simulink model "MRAC_OutputFeedback_Tau"  (R2017b)
settings: Solver=VariableStepAuto  StartTime=0.0  StopTime=100  RelTol=1e-3
values from neighbouring files (symbols this model uses):
  Ix = 0.0552    [ProportionalController.m]    (also in discrete1.m; discrete2.m; istr.m; proportionalTest.m = 0.0235)
  Iy = 0.0552    [ProportionalController.m]    (also in discrete1.m; discrete2.m; istr.m; proportionalTest.m = 0.0494)
  Iz = 0.11    [ProportionalController.m]    (also in discrete1.m; discrete2.m; istr.m; proportionalTest.m = 0.6121)
  wn = 4/(zeta*Ts)    [SecondOrderResponse.m]
  zeta = 0.7    [RLS_demo_init.m]    (also in SecondOrderResponse.m = sqrt(A/(pi^2+A)))
undefined symbols (not defined in the file or in its folder): a0, b0_zero_p, b0_zero_r, b0_zero_y, DiscIntNeverNeededParam, gamma1_p, gamma1_r, gamma1_y, gamma2_p, gamma2_r, gamma2_y, theta_zero_p, theta_zero_r, theta_zero_y
libraries: simulink_extras x15
settings Model: Creator=YvesDaoud  LastModifiedBy=YvesDaoud

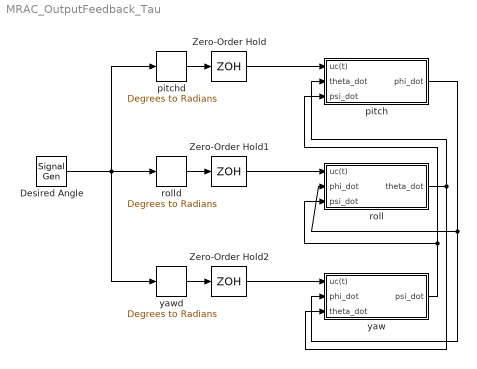
== system MRAC_OutputFeedback_Tau ==
  Desired Angle : SignalGenerator  WaveForm=square  Amplitude=5  Frequency=0.05
  Zero-Order Hold : ZeroOrderHold  SampleTime=1/2000
  Zero-Order Hold1 : ZeroOrderHold  SampleTime=1/2000
  Zero-Order Hold2 : ZeroOrderHold  SampleTime=1/2000
  pitch : Subsystem
  pitchd : simulink_extras/Transformations/Degrees to Radians
  roll : Subsystem
  rolld : simulink_extras/Transformations/Degrees to Radians
  yaw : Subsystem
  yawd : simulink_extras/Transformations/Degrees to Radians
  wires:
  rolld/1 -> Zero-Order Hold1/1
  yawd/1 -> Zero-Order Hold2/1
  Zero-Order Hold/1 -> pitch/1(uc(t))
  Zero-Order Hold1/1 -> roll/1(uc(t))
  Desired Angle/1 -> pitchd/1, yawd/1, rolld/1
  pitchd/1 -> Zero-Order Hold/1
  Zero-Order Hold2/1 -> yaw/1(uc(t))
  roll/1(theta_dot) -> yaw/3(theta_dot), pitch/2(theta_dot)
  pitch/1(phi_dot) -> roll/2(phi_dot), yaw/2(phi_dot)
  yaw/1(psi_dot) -> roll/3(psi_dot), pitch/3(psi_dot)

== system MRAC_OutputFeedback_Tau/pitch ==
  uc(t) : Inport
  theta_dot : Inport  Port=2
  psi_dot : Inport  Port=3
  Controller : Subsystem
  Plant : Subsystem
  Plotting : Subsystem
  Reference Model : Subsystem
  augmented error : Subsystem
  b0_hat : Subsystem
  eta n : Subsystem
  theta : Subsystem
  phi_dot : Outport
  wires:
  Plant/1(y(t)) -> Plotting/2(y(t)), theta/3(y(t)), Controller/2(y(t)), augmented error/1(y(t)), eta n/2(y(t))
  Reference Model/1(ym(t)) -> Plotting/3(ym(t)), augmented error/2(ym(t))
  Controller/1(u(t)) -> Plant/1(u(t)), Plotting/4(u(t)), eta n/1(u(t)), theta/2(u(t))
  theta/1(theta) -> Controller/3(theta), eta n/4(theta)
  eta n/1(eta n) -> b0_hat/1(eta n), augmented error/4(eta n)
  b0_hat/1(b0_hat) -> Plotting/5(b0_hat), augmented error/3(b0_hat)
  uc(t)/1 -> Plotting/1(uc(t)), theta/4(uc(t)), Reference Model/1(uc(t)), eta n/3(uc(t)), Controller/1(uc(t))
  augmented error/1(epsilon) -> b0_hat/2(epsilon), theta/1(epsilon)
  theta_dot/1 -> Plant/2(theta_dot)
  psi_dot/1 -> Plant/3(psi_dot)
  Plant/2(y_dot(t)) -> phi_dot/1

== system MRAC_OutputFeedback_Tau/roll ==
  uc(t) : Inport
  phi_dot : Inport  Port=2
  psi_dot : Inport  Port=3
  Controller : Subsystem
  Plant : Subsystem
  Plotting : Subsystem
  Reference Model : Subsystem
  augmented error : Subsystem
  b0_hat : Subsystem
  eta n : Subsystem
  theta : Subsystem
  theta_dot : Outport
  wires:
  Plant/2(y_dot(t)) -> theta_dot/1
  psi_dot/1 -> Plant/3(psi_dot)
  phi_dot/1 -> Plant/2(phi_dot)
  augmented error/1(epsilon) -> theta/1(epsilon), b0_hat/2(epsilon)
  uc(t)/1 -> Controller/1(uc(t)), eta n/3(uc(t)), Reference Model/1(uc(t)), theta/4(uc(t)), Plotting/1(uc(t))
  b0_hat/1(b0_hat) -> augmented error/3(b0_hat), Plotting/5(b0_hat)
  eta n/1(eta n) -> augmented error/4(eta n), b0_hat/1(eta n)
  theta/1(theta) -> eta n/4(theta), Controller/3(theta)
  Controller/1(u(t)) -> theta/2(u(t)), eta n/1(u(t)), Plotting/4(u(t)), Plant/1(u(t))
  Reference Model/1(ym(t)) -> augmented error/2(ym(t)), Plotting/3(ym(t))
  Plant/1(y(t)) -> eta n/2(y(t)), augmented error/1(y(t)), Controller/2(y(t)), theta/3(y(t)), Plotting/2(y(t))

== system MRAC_OutputFeedback_Tau/yaw ==
  uc(t) : Inport
  phi_dot : Inport  Port=2
  theta_dot : Inport  Port=3
  Controller : Subsystem
  Plant : Subsystem
  Plotting : Subsystem
  Reference Model : Subsystem
  augmented error : Subsystem
  b0_hat : Subsystem
  eta n : Subsystem
  theta : Subsystem
  psi_dot : Outport
  wires:
  Plant/1(y(t)) -> Plotting/2(y(t)), theta/3(y(t)), Controller/2(y(t)), augmented error/1(y(t)), eta n/2(y(t))
  Reference Model/1(ym(t)) -> Plotting/3(ym(t)), augmented error/2(ym(t))
  Controller/1(u(t)) -> Plant/1(u(t)), Plotting/4(u(t)), eta n/1(u(t)), theta/2(u(t))
  theta/1(theta) -> Controller/3(theta), eta n/4(theta)
  eta n/1(eta n) -> b0_hat/1(eta n), augmented error/4(eta n)
  b0_hat/1(b0_hat) -> Plotting/5(b0_hat), augmented error/3(b0_hat)
  uc(t)/1 -> Plotting/1(uc(t)), theta/4(uc(t)), Reference Model/1(uc(t)), eta n/3(uc(t)), Controller/1(uc(t))
  augmented error/1(epsilon) -> b0_hat/2(epsilon), theta/1(epsilon)
  phi_dot/1 -> Plant/2(phi_dot)
  theta_dot/1 -> Plant/3(theta_dot)
  Plant/2(y_dot(t)) -> psi_dot/1

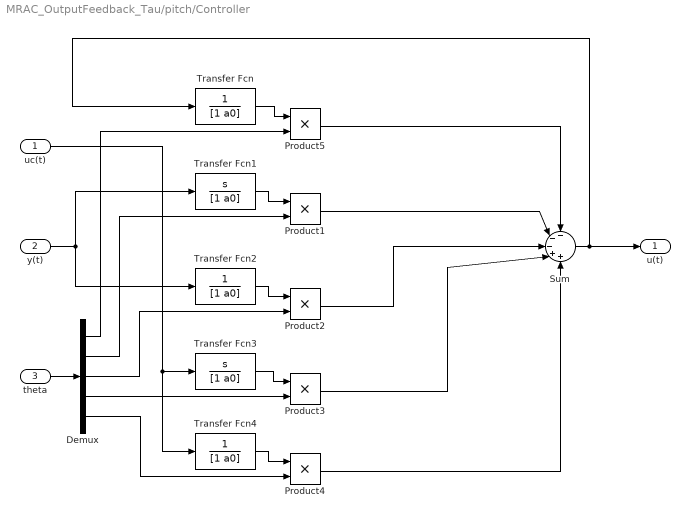
== system MRAC_OutputFeedback_Tau/pitch/Controller ==
  uc(t) : Inport
  y(t) : Inport  Port=2
  theta : Inport  Port=3
  Demux : Demux  Outputs=5
  Product{1..5} (5 alike) : Product
  Sum : Sum  Inputs=---++
  Transfer Fcn : TransferFcn  Denominator=[1 a0]
  Transfer Fcn1 : TransferFcn  Numerator=[1 0]  Denominator=[1 a0]
  Transfer Fcn2 : TransferFcn  Denominator=[1 a0]
  Transfer Fcn3 : TransferFcn  Numerator=[1 0]  Denominator=[1 a0]
  Transfer Fcn4 : TransferFcn  Denominator=[1 a0]
  u(t) : Outport
  wires:
  theta/1 -> Demux/1
  Transfer Fcn1/1 -> Product1/1
  Transfer Fcn2/1 -> Product2/1
  Transfer Fcn3/1 -> Product3/1
  Transfer Fcn4/1 -> Product4/1
  Transfer Fcn/1 -> Product5/1
  Sum/1 -> u(t)/1, Transfer Fcn/1
  Demux/1 -> Product5/2
  Product5/1 -> Sum/1
  Product1/1 -> Sum/2
  Product2/1 -> Sum/3
  Product3/1 -> Sum/4
  Product4/1 -> Sum/5
  y(t)/1 -> Transfer Fcn2/1, Transfer Fcn1/1
  Demux/2 -> Product1/2
  Demux/3 -> Product2/2
  Demux/4 -> Product3/2
  uc(t)/1 -> Transfer Fcn4/1, Transfer Fcn3/1
  Demux/5 -> Product4/2

== system MRAC_OutputFeedback_Tau/pitch/Plant ==
  u(t) : Inport
  theta_dot : Inport  Port=2
  psi_dot : Inport  Port=3
  Constant : Constant  Value=(Iy-Iz)/Ix
  Constant1 : Constant  Value=1/Ix
  Integrator : Integrator
  Integrator1 : Integrator
  Product : Product  Inputs=3
  Product1 : Product
  Sum : Sum  Inputs=+|+
  y(t) : Outport
  y_dot(t) : Outport  Port=2
  wires:
  u(t)/1 -> Product1/1
  Integrator/1 -> y_dot(t)/1, Integrator1/1
  Integrator1/1 -> y(t)/1
  theta_dot/1 -> Product/2
  Product1/1 -> Sum/1
  Constant1/1 -> Product1/2
  Constant/1 -> Product/1
  Product/1 -> Sum/2
  Sum/1 -> Integrator/1
  psi_dot/1 -> Product/3

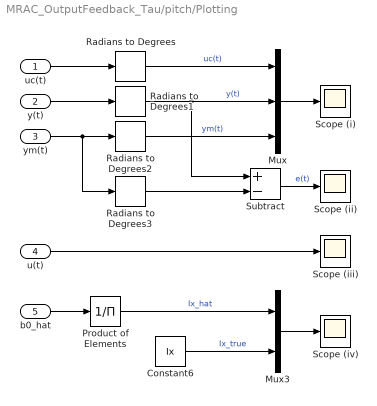
== system MRAC_OutputFeedback_Tau/pitch/Plotting ==
  uc(t) : Inport
  y(t) : Inport  Port=2
  ym(t) : Inport  Port=3
  u(t) : Inport  Port=4
  b0_hat : Inport  Port=5
  Constant6 : Constant  Value=Ix
  Mux : Mux  Inputs=3
  Mux3 : Mux  Inputs=2
  Product of Elements : Product  Inputs=/
  Radians to Degrees{,1..3} (4 alike) : simulink_extras/Transformations/Radians to Degrees
  Scope (i) : Scope
  Scope (ii) : Scope
  Scope (iii) : Scope
  Scope (iv) : Scope
  Subtract : Sum  Inputs=+-
  wires:
  u(t)/1 -> Scope (iii)/1
  b0_hat/1 -> Product of Elements/1
  Mux3/1 -> Scope (iv)/1
  Product of Elements/1 -> Mux3/1  "Ix_hat"
  Constant6/1 -> Mux3/2  "Ix_true"
  Subtract/1 -> Scope (ii)/1  "e(t)"
  uc(t)/1 -> Radians to Degrees/1
  y(t)/1 -> Radians to Degrees1/1
  Mux/1 -> Scope (i)/1
  Radians to Degrees/1 -> Mux/1  "uc(t)"
  Radians to Degrees2/1 -> Mux/3  "ym(t)"
  ym(t)/1 -> Radians to Degrees3/1, Radians to Degrees2/1
  Radians to Degrees1/1 -> Subtract/1, Mux/2  "y(t)"
  Radians to Degrees3/1 -> Subtract/2

== system MRAC_OutputFeedback_Tau/pitch/Reference Model ==
  uc(t) : Inport
  Transfer Fcn11 : TransferFcn  Numerator=[wn^2]  Denominator=[1 2*zeta*wn wn^2]
  ym(t) : Outport
  wires:
  uc(t)/1 -> Transfer Fcn11/1
  Transfer Fcn11/1 -> ym(t)/1

== system MRAC_OutputFeedback_Tau/pitch/augmented error ==
  y(t) : Inport
  ym(t) : Inport  Port=2
  b0_hat : Inport  Port=3
  eta n : Inport  Port=4
  Product : Product
  Sum : Sum  Inputs=+-+
  epsilon : Outport
  wires:
  b0_hat/1 -> Product/1
  eta n/1 -> Product/2
  y(t)/1 -> Sum/1
  ym(t)/1 -> Sum/2
  Product/1 -> Sum/3
  Sum/1 -> epsilon/1

== system MRAC_OutputFeedback_Tau/pitch/b0_hat ==
  eta n : Inport
  epsilon : Inport  Port=2
  Discrete-Time Integrator : DiscreteIntegrator  InitialCondition=b0_zero_p  InitialConditionSetting=State (most efficient)  SampleTime=-1  ICPrevOutput=DiscIntNeverNeededParam  ICPrevScaledInput=DiscIntNeverNeededParam
  Gain : Gain  Gain=-1
  Product : Product  Inputs=3
  gamma1 : Constant  Value=gamma1_p
  b0_hat : Outport
  wires:
  gamma1/1 -> Gain/1
  eta n/1 -> Product/2
  Gain/1 -> Product/1
  epsilon/1 -> Product/3
  Product/1 -> Discrete-Time Integrator/1
  Discrete-Time Integrator/1 -> b0_hat/1

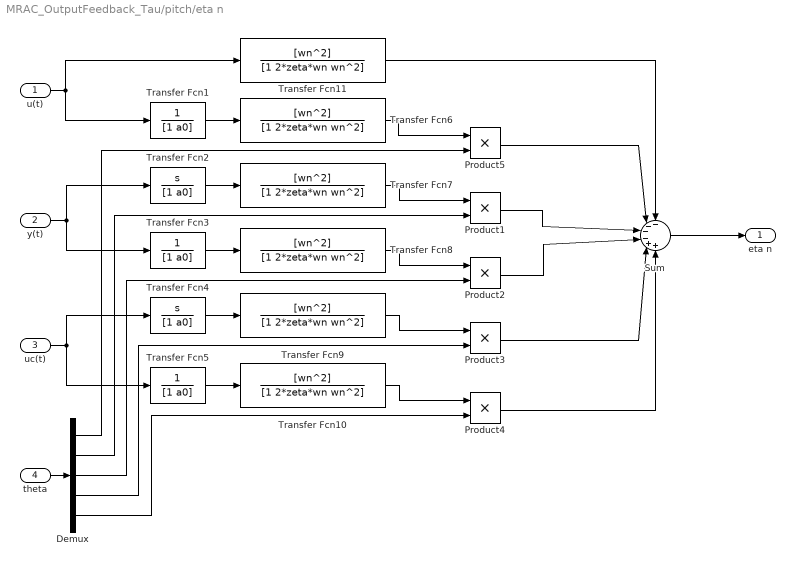
== system MRAC_OutputFeedback_Tau/pitch/eta n ==
  u(t) : Inport
  y(t) : Inport  Port=2
  uc(t) : Inport  Port=3
  theta : Inport  Port=4
  Demux : Demux  Outputs=5
  Product{1..5} (5 alike) : Product
  Sum : Sum  Inputs=----++
  Transfer Fcn1 : TransferFcn  Denominator=[1 a0]
  Transfer Fcn{6..11} (6 alike) : TransferFcn  Numerator=[wn^2]  Denominator=[1 2*zeta*wn wn^2]
  Transfer Fcn2 : TransferFcn  Numerator=[1 0]  Denominator=[1 a0]
  Transfer Fcn3 : TransferFcn  Denominator=[1 a0]
  Transfer Fcn4 : TransferFcn  Numerator=[1 0]  Denominator=[1 a0]
  Transfer Fcn5 : TransferFcn  Denominator=[1 a0]
  eta n : Outport
  wires:
  theta/1 -> Demux/1
  Transfer Fcn11/1 -> Sum/1
  u(t)/1 -> Transfer Fcn11/1, Transfer Fcn1/1
  Sum/1 -> eta n/1
  Demux/1 -> Product5/2
  Demux/2 -> Product1/2
  Demux/3 -> Product2/2
  Demux/4 -> Product3/2
  Demux/5 -> Product4/2
  y(t)/1 -> Transfer Fcn3/1, Transfer Fcn2/1
  uc(t)/1 -> Transfer Fcn5/1, Transfer Fcn4/1
  Product5/1 -> Sum/2
  Product1/1 -> Sum/3
  Product2/1 -> Sum/4
  Product3/1 -> Sum/5
  Product4/1 -> Sum/6
  Transfer Fcn1/1 -> Transfer Fcn6/1
  Transfer Fcn6/1 -> Product5/1
  Transfer Fcn2/1 -> Transfer Fcn7/1
  Transfer Fcn7/1 -> Product1/1
  Transfer Fcn3/1 -> Transfer Fcn8/1
  Transfer Fcn8/1 -> Product2/1
  Transfer Fcn4/1 -> Transfer Fcn9/1
  Transfer Fcn9/1 -> Product3/1
  Transfer Fcn5/1 -> Transfer Fcn10/1
  Transfer Fcn10/1 -> Product4/1

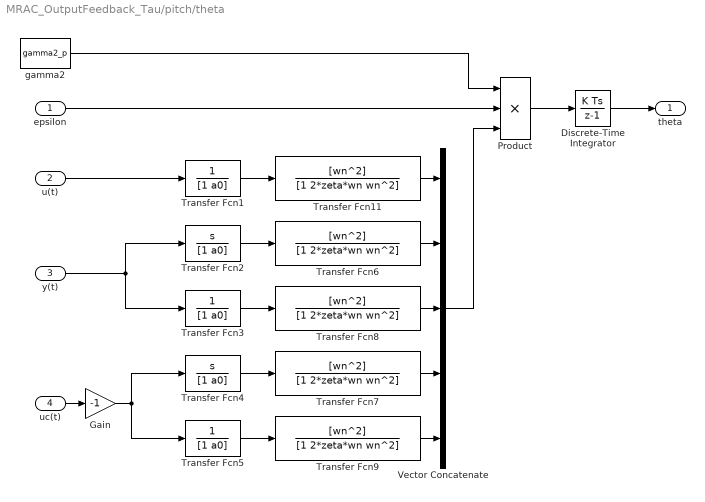
== system MRAC_OutputFeedback_Tau/pitch/theta ==
  epsilon : Inport
  u(t) : Inport  Port=2
  y(t) : Inport  Port=3
  uc(t) : Inport  Port=4
  Discrete-Time Integrator : DiscreteIntegrator  InitialCondition=theta_zero_p  InitialConditionSetting=State (most efficient)  SampleTime=-1  ICPrevOutput=DiscIntNeverNeededParam  ICPrevScaledInput=DiscIntNeverNeededParam
  Gain : Gain  Gain=-1
  Product : Product  Inputs=3
  Transfer Fcn1 : TransferFcn  Denominator=[1 a0]
  Transfer Fcn{6..9,11} (5 alike) : TransferFcn  Numerator=[wn^2]  Denominator=[1 2*zeta*wn wn^2]
  Transfer Fcn2 : TransferFcn  Numerator=[1 0]  Denominator=[1 a0]
  Transfer Fcn3 : TransferFcn  Denominator=[1 a0]
  Transfer Fcn4 : TransferFcn  Numerator=[1 0]  Denominator=[1 a0]
  Transfer Fcn5 : TransferFcn  Denominator=[1 a0]
  Vector Concatenate : Concatenate  NumInputs=5
  gamma2 : Constant  Value=gamma2_p
  theta : Outport
  wires:
  gamma2/1 -> Product/1
  epsilon/1 -> Product/2
  Discrete-Time Integrator/1 -> theta/1
  Product/1 -> Discrete-Time Integrator/1
  Transfer Fcn2/1 -> Transfer Fcn6/1
  Transfer Fcn4/1 -> Transfer Fcn7/1
  Transfer Fcn3/1 -> Transfer Fcn8/1
  Transfer Fcn5/1 -> Transfer Fcn9/1
  Transfer Fcn1/1 -> Transfer Fcn11/1
  u(t)/1 -> Transfer Fcn1/1
  Transfer Fcn9/1 -> Vector Concatenate/5
  Transfer Fcn7/1 -> Vector Concatenate/4
  Transfer Fcn8/1 -> Vector Concatenate/3
  Transfer Fcn6/1 -> Vector Concatenate/2
  Transfer Fcn11/1 -> Vector Concatenate/1
  y(t)/1 -> Transfer Fcn2/1, Transfer Fcn3/1
  uc(t)/1 -> Gain/1
  Gain/1 -> Transfer Fcn5/1, Transfer Fcn4/1
  Vector Concatenate/1 -> Product/3

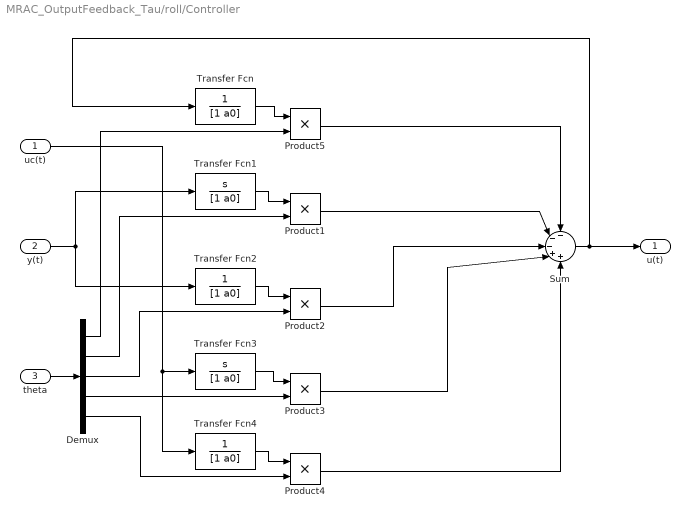
== system MRAC_OutputFeedback_Tau/roll/Controller ==
  uc(t) : Inport
  y(t) : Inport  Port=2
  theta : Inport  Port=3
  Demux : Demux  Outputs=5
  Product{1..5} (5 alike) : Product
  Sum : Sum  Inputs=---++
  Transfer Fcn : TransferFcn  Denominator=[1 a0]
  Transfer Fcn1 : TransferFcn  Numerator=[1 0]  Denominator=[1 a0]
  Transfer Fcn2 : TransferFcn  Denominator=[1 a0]
  Transfer Fcn3 : TransferFcn  Numerator=[1 0]  Denominator=[1 a0]
  Transfer Fcn4 : TransferFcn  Denominator=[1 a0]
  u(t) : Outport
  wires:
  Demux/5 -> Product4/2
  uc(t)/1 -> Transfer Fcn3/1, Transfer Fcn4/1
  Demux/4 -> Product3/2
  Demux/3 -> Product2/2
  Demux/2 -> Product1/2
  y(t)/1 -> Transfer Fcn1/1, Transfer Fcn2/1
  Product4/1 -> Sum/5
  Product3/1 -> Sum/4
  Product2/1 -> Sum/3
  Product1/1 -> Sum/2
  Product5/1 -> Sum/1
  Demux/1 -> Product5/2
  Sum/1 -> Transfer Fcn/1, u(t)/1
  Transfer Fcn/1 -> Product5/1
  Transfer Fcn4/1 -> Product4/1
  Transfer Fcn3/1 -> Product3/1
  Transfer Fcn2/1 -> Product2/1
  Transfer Fcn1/1 -> Product1/1
  theta/1 -> Demux/1

== system MRAC_OutputFeedback_Tau/roll/Plant ==
  u(t) : Inport
  phi_dot : Inport  Port=2
  psi_dot : Inport  Port=3
  Constant : Constant  Value=(Iz-Ix)/Iy
  Constant1 : Constant  Value=1/Iy
  Integrator : Integrator
  Integrator1 : Integrator
  Product : Product  Inputs=3
  Product1 : Product
  Sum : Sum  Inputs=+|+
  y(t) : Outport
  y_dot(t) : Outport  Port=2
  wires:
  psi_dot/1 -> Product/3
  Sum/1 -> Integrator/1
  Product/1 -> Sum/2
  Constant/1 -> Product/1
  Constant1/1 -> Product1/2
  Product1/1 -> Sum/1
  phi_dot/1 -> Product/2
  Integrator1/1 -> y(t)/1
  Integrator/1 -> Integrator1/1, y_dot(t)/1
  u(t)/1 -> Product1/1

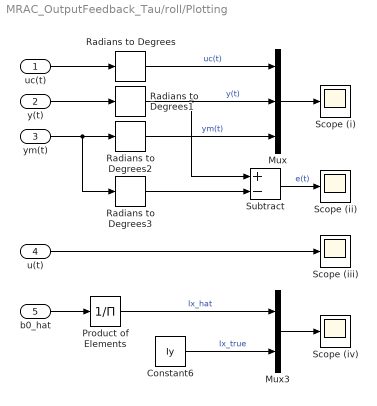
== system MRAC_OutputFeedback_Tau/roll/Plotting ==
  uc(t) : Inport
  y(t) : Inport  Port=2
  ym(t) : Inport  Port=3
  u(t) : Inport  Port=4
  b0_hat : Inport  Port=5
  Constant6 : Constant  Value=Iy
  Mux : Mux  Inputs=3
  Mux3 : Mux  Inputs=2
  Product of Elements : Product  Inputs=/
  Radians to Degrees{,1..3} (4 alike) : simulink_extras/Transformations/Radians to Degrees
  Scope (i) : Scope
  Scope (ii) : Scope
  Scope (iii) : Scope
  Scope (iv) : Scope
  Subtract : Sum  Inputs=+-
  wires:
  Radians to Degrees3/1 -> Subtract/2
  Radians to Degrees1/1 -> Mux/2, Subtract/1  "y(t)"
  ym(t)/1 -> Radians to Degrees2/1, Radians to Degrees3/1
  Radians to Degrees2/1 -> Mux/3  "ym(t)"
  Radians to Degrees/1 -> Mux/1  "uc(t)"
  Mux/1 -> Scope (i)/1
  y(t)/1 -> Radians to Degrees1/1
  uc(t)/1 -> Radians to Degrees/1
  Subtract/1 -> Scope (ii)/1  "e(t)"
  Constant6/1 -> Mux3/2  "Ix_true"
  Product of Elements/1 -> Mux3/1  "Ix_hat"
  Mux3/1 -> Scope (iv)/1
  b0_hat/1 -> Product of Elements/1
  u(t)/1 -> Scope (iii)/1

== system MRAC_OutputFeedback_Tau/roll/Reference Model ==
  uc(t) : Inport
  Transfer Fcn11 : TransferFcn  Numerator=[wn^2]  Denominator=[1 2*zeta*wn wn^2]
  ym(t) : Outport
  wires:
  Transfer Fcn11/1 -> ym(t)/1
  uc(t)/1 -> Transfer Fcn11/1

== system MRAC_OutputFeedback_Tau/roll/augmented error ==
  y(t) : Inport
  ym(t) : Inport  Port=2
  b0_hat : Inport  Port=3
  eta n : Inport  Port=4
  Product : Product
  Sum : Sum  Inputs=+-+
  epsilon : Outport
  wires:
  Sum/1 -> epsilon/1
  Product/1 -> Sum/3
  ym(t)/1 -> Sum/2
  y(t)/1 -> Sum/1
  eta n/1 -> Product/2
  b0_hat/1 -> Product/1

== system MRAC_OutputFeedback_Tau/roll/b0_hat ==
  eta n : Inport
  epsilon : Inport  Port=2
  Discrete-Time Integrator : DiscreteIntegrator  InitialCondition=b0_zero_r  InitialConditionSetting=State (most efficient)  SampleTime=-1  ICPrevOutput=DiscIntNeverNeededParam  ICPrevScaledInput=DiscIntNeverNeededParam
  Gain : Gain  Gain=-1
  Product : Product  Inputs=3
  gamma1 : Constant  Value=gamma1_r
  b0_hat : Outport
  wires:
  Discrete-Time Integrator/1 -> b0_hat/1
  Product/1 -> Discrete-Time Integrator/1
  epsilon/1 -> Product/3
  Gain/1 -> Product/1
  eta n/1 -> Product/2
  gamma1/1 -> Gain/1

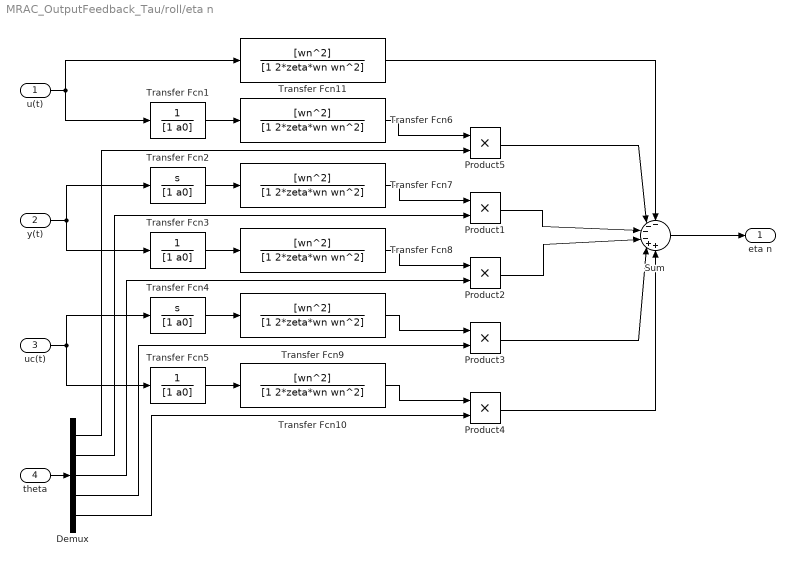
== system MRAC_OutputFeedback_Tau/roll/eta n ==
  u(t) : Inport
  y(t) : Inport  Port=2
  uc(t) : Inport  Port=3
  theta : Inport  Port=4
  Demux : Demux  Outputs=5
  Product{1..5} (5 alike) : Product
  Sum : Sum  Inputs=----++
  Transfer Fcn1 : TransferFcn  Denominator=[1 a0]
  Transfer Fcn{6..11} (6 alike) : TransferFcn  Numerator=[wn^2]  Denominator=[1 2*zeta*wn wn^2]
  Transfer Fcn2 : TransferFcn  Numerator=[1 0]  Denominator=[1 a0]
  Transfer Fcn3 : TransferFcn  Denominator=[1 a0]
  Transfer Fcn4 : TransferFcn  Numerator=[1 0]  Denominator=[1 a0]
  Transfer Fcn5 : TransferFcn  Denominator=[1 a0]
  eta n : Outport
  wires:
  Transfer Fcn10/1 -> Product4/1
  Transfer Fcn5/1 -> Transfer Fcn10/1
  Transfer Fcn9/1 -> Product3/1
  Transfer Fcn4/1 -> Transfer Fcn9/1
  Transfer Fcn8/1 -> Product2/1
  Transfer Fcn3/1 -> Transfer Fcn8/1
  Transfer Fcn7/1 -> Product1/1
  Transfer Fcn2/1 -> Transfer Fcn7/1
  Transfer Fcn6/1 -> Product5/1
  Transfer Fcn1/1 -> Transfer Fcn6/1
  Product4/1 -> Sum/6
  Product3/1 -> Sum/5
  Product2/1 -> Sum/4
  Product1/1 -> Sum/3
  Product5/1 -> Sum/2
  uc(t)/1 -> Transfer Fcn4/1, Transfer Fcn5/1
  y(t)/1 -> Transfer Fcn2/1, Transfer Fcn3/1
  Demux/5 -> Product4/2
  Demux/4 -> Product3/2
  Demux/3 -> Product2/2
  Demux/2 -> Product1/2
  Demux/1 -> Product5/2
  Sum/1 -> eta n/1
  u(t)/1 -> Transfer Fcn1/1, Transfer Fcn11/1
  Transfer Fcn11/1 -> Sum/1
  theta/1 -> Demux/1

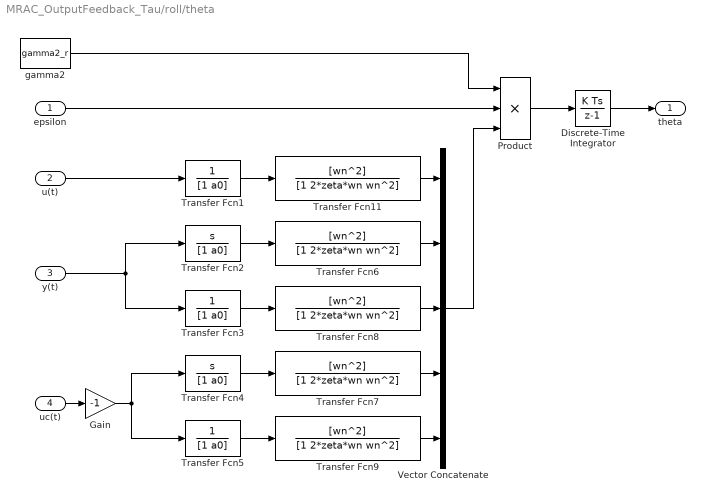
== system MRAC_OutputFeedback_Tau/roll/theta ==
  epsilon : Inport
  u(t) : Inport  Port=2
  y(t) : Inport  Port=3
  uc(t) : Inport  Port=4
  Discrete-Time Integrator : DiscreteIntegrator  InitialCondition=theta_zero_r  InitialConditionSetting=State (most efficient)  SampleTime=-1  ICPrevOutput=DiscIntNeverNeededParam  ICPrevScaledInput=DiscIntNeverNeededParam
  Gain : Gain  Gain=-1
  Product : Product  Inputs=3
  Transfer Fcn1 : TransferFcn  Denominator=[1 a0]
  Transfer Fcn{6..9,11} (5 alike) : TransferFcn  Numerator=[wn^2]  Denominator=[1 2*zeta*wn wn^2]
  Transfer Fcn2 : TransferFcn  Numerator=[1 0]  Denominator=[1 a0]
  Transfer Fcn3 : TransferFcn  Denominator=[1 a0]
  Transfer Fcn4 : TransferFcn  Numerator=[1 0]  Denominator=[1 a0]
  Transfer Fcn5 : TransferFcn  Denominator=[1 a0]
  Vector Concatenate : Concatenate  NumInputs=5
  gamma2 : Constant  Value=gamma2_r
  theta : Outport
  wires:
  Vector Concatenate/1 -> Product/3
  Gain/1 -> Transfer Fcn4/1, Transfer Fcn5/1
  uc(t)/1 -> Gain/1
  y(t)/1 -> Transfer Fcn3/1, Transfer Fcn2/1
  Transfer Fcn11/1 -> Vector Concatenate/1
  Transfer Fcn6/1 -> Vector Concatenate/2
  Transfer Fcn8/1 -> Vector Concatenate/3
  Transfer Fcn7/1 -> Vector Concatenate/4
  Transfer Fcn9/1 -> Vector Concatenate/5
  u(t)/1 -> Transfer Fcn1/1
  Transfer Fcn1/1 -> Transfer Fcn11/1
  Transfer Fcn5/1 -> Transfer Fcn9/1
  Transfer Fcn3/1 -> Transfer Fcn8/1
  Transfer Fcn4/1 -> Transfer Fcn7/1
  Transfer Fcn2/1 -> Transfer Fcn6/1
  Product/1 -> Discrete-Time Integrator/1
  Discrete-Time Integrator/1 -> theta/1
  epsilon/1 -> Product/2
  gamma2/1 -> Product/1

== system MRAC_OutputFeedback_Tau/yaw/Controller ==
  uc(t) : Inport
  y(t) : Inport  Port=2
  theta : Inport  Port=3
  Demux : Demux  Outputs=5
  Product{1..5} (5 alike) : Product
  Sum : Sum  Inputs=---++
  Transfer Fcn : TransferFcn  Denominator=[1 a0]
  Transfer Fcn1 : TransferFcn  Numerator=[1 0]  Denominator=[1 a0]
  Transfer Fcn2 : TransferFcn  Denominator=[1 a0]
  Transfer Fcn3 : TransferFcn  Numerator=[1 0]  Denominator=[1 a0]
  Transfer Fcn4 : TransferFcn  Denominator=[1 a0]
  u(t) : Outport
  wires:
  theta/1 -> Demux/1
  Transfer Fcn1/1 -> Product1/1
  Transfer Fcn2/1 -> Product2/1
  Transfer Fcn3/1 -> Product3/1
  Transfer Fcn4/1 -> Product4/1
  Transfer Fcn/1 -> Product5/1
  Sum/1 -> u(t)/1, Transfer Fcn/1
  Demux/1 -> Product5/2
  Product5/1 -> Sum/1
  Product1/1 -> Sum/2
  Product2/1 -> Sum/3
  Product3/1 -> Sum/4
  Product4/1 -> Sum/5
  y(t)/1 -> Transfer Fcn2/1, Transfer Fcn1/1
  Demux/2 -> Product1/2
  Demux/3 -> Product2/2
  Demux/4 -> Product3/2
  uc(t)/1 -> Transfer Fcn4/1, Transfer Fcn3/1
  Demux/5 -> Product4/2

== system MRAC_OutputFeedback_Tau/yaw/Plant ==
  u(t) : Inport
  phi_dot : Inport  Port=2
  theta_dot : Inport  Port=3
  Constant : Constant  Value=(Ix-Iy)/Iz
  Constant1 : Constant  Value=1/Iz
  Integrator : Integrator
  Integrator1 : Integrator
  Product : Product  Inputs=3
  Product1 : Product
  Sum : Sum  Inputs=+|+
  y(t) : Outport
  y_dot(t) : Outport  Port=2
  wires:
  u(t)/1 -> Product1/1
  Integrator/1 -> y_dot(t)/1, Integrator1/1
  Integrator1/1 -> y(t)/1
  phi_dot/1 -> Product/2
  Product1/1 -> Sum/1
  Constant1/1 -> Product1/2
  Constant/1 -> Product/1
  Product/1 -> Sum/2
  Sum/1 -> Integrator/1
  theta_dot/1 -> Product/3

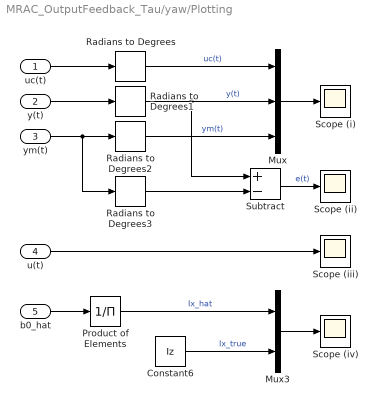
== system MRAC_OutputFeedback_Tau/yaw/Plotting ==
  uc(t) : Inport
  y(t) : Inport  Port=2
  ym(t) : Inport  Port=3
  u(t) : Inport  Port=4
  b0_hat : Inport  Port=5
  Constant6 : Constant  Value=Iz
  Mux : Mux  Inputs=3
  Mux3 : Mux  Inputs=2
  Product of Elements : Product  Inputs=/
  Radians to Degrees{,1..3} (4 alike) : simulink_extras/Transformations/Radians to Degrees
  Scope (i) : Scope
  Scope (ii) : Scope
  Scope (iii) : Scope
  Scope (iv) : Scope
  Subtract : Sum  Inputs=+-
  wires:
  u(t)/1 -> Scope (iii)/1
  b0_hat/1 -> Product of Elements/1
  Mux3/1 -> Scope (iv)/1
  Product of Elements/1 -> Mux3/1  "Ix_hat"
  Constant6/1 -> Mux3/2  "Ix_true"
  Subtract/1 -> Scope (ii)/1  "e(t)"
  uc(t)/1 -> Radians to Degrees/1
  y(t)/1 -> Radians to Degrees1/1
  Mux/1 -> Scope (i)/1
  Radians to Degrees/1 -> Mux/1  "uc(t)"
  Radians to Degrees2/1 -> Mux/3  "ym(t)"
  ym(t)/1 -> Radians to Degrees3/1, Radians to Degrees2/1
  Radians to Degrees1/1 -> Subtract/1, Mux/2  "y(t)"
  Radians to Degrees3/1 -> Subtract/2

== system MRAC_OutputFeedback_Tau/yaw/Reference Model ==
  uc(t) : Inport
  Transfer Fcn11 : TransferFcn  Numerator=[wn^2]  Denominator=[1 2*zeta*wn wn^2]
  ym(t) : Outport
  wires:
  uc(t)/1 -> Transfer Fcn11/1
  Transfer Fcn11/1 -> ym(t)/1

== system MRAC_OutputFeedback_Tau/yaw/augmented error ==
  y(t) : Inport
  ym(t) : Inport  Port=2
  b0_hat : Inport  Port=3
  eta n : Inport  Port=4
  Product : Product
  Sum : Sum  Inputs=+-+
  epsilon : Outport
  wires:
  b0_hat/1 -> Product/1
  eta n/1 -> Product/2
  y(t)/1 -> Sum/1
  ym(t)/1 -> Sum/2
  Product/1 -> Sum/3
  Sum/1 -> epsilon/1

== system MRAC_OutputFeedback_Tau/yaw/b0_hat ==
  eta n : Inport
  epsilon : Inport  Port=2
  Discrete-Time Integrator : DiscreteIntegrator  InitialCondition=b0_zero_y  InitialConditionSetting=State (most efficient)  SampleTime=-1  ICPrevOutput=DiscIntNeverNeededParam  ICPrevScaledInput=DiscIntNeverNeededParam
  Gain : Gain  Gain=-1
  Product : Product  Inputs=3
  gamma1 : Constant  Value=gamma1_y
  b0_hat : Outport
  wires:
  gamma1/1 -> Gain/1
  eta n/1 -> Product/2
  Gain/1 -> Product/1
  epsilon/1 -> Product/3
  Product/1 -> Discrete-Time Integrator/1
  Discrete-Time Integrator/1 -> b0_hat/1

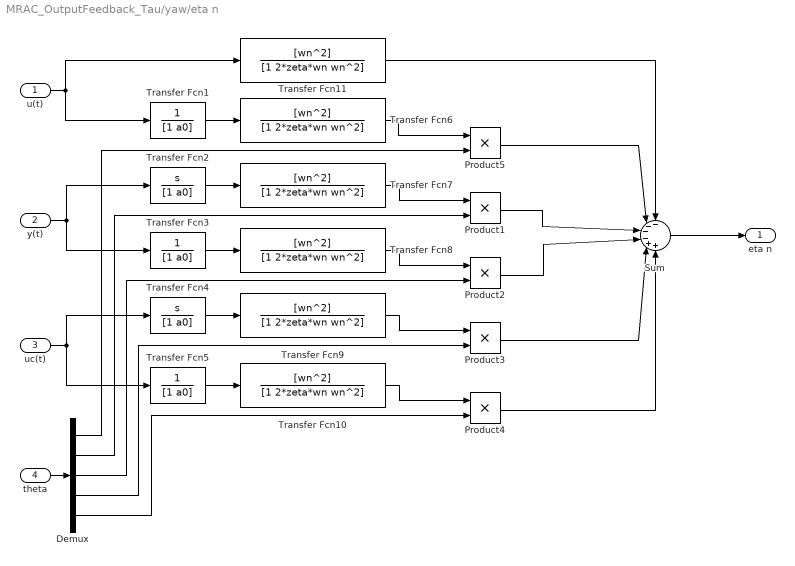
== system MRAC_OutputFeedback_Tau/yaw/eta n ==
  u(t) : Inport
  y(t) : Inport  Port=2
  uc(t) : Inport  Port=3
  theta : Inport  Port=4
  Demux : Demux  Outputs=5
  Product{1..5} (5 alike) : Product
  Sum : Sum  Inputs=----++
  Transfer Fcn1 : TransferFcn  Denominator=[1 a0]
  Transfer Fcn{6..11} (6 alike) : TransferFcn  Numerator=[wn^2]  Denominator=[1 2*zeta*wn wn^2]
  Transfer Fcn2 : TransferFcn  Numerator=[1 0]  Denominator=[1 a0]
  Transfer Fcn3 : TransferFcn  Denominator=[1 a0]
  Transfer Fcn4 : TransferFcn  Numerator=[1 0]  Denominator=[1 a0]
  Transfer Fcn5 : TransferFcn  Denominator=[1 a0]
  eta n : Outport
  wires:
  theta/1 -> Demux/1
  Transfer Fcn11/1 -> Sum/1
  u(t)/1 -> Transfer Fcn11/1, Transfer Fcn1/1
  Sum/1 -> eta n/1
  Demux/1 -> Product5/2
  Demux/2 -> Product1/2
  Demux/3 -> Product2/2
  Demux/4 -> Product3/2
  Demux/5 -> Product4/2
  y(t)/1 -> Transfer Fcn3/1, Transfer Fcn2/1
  uc(t)/1 -> Transfer Fcn5/1, Transfer Fcn4/1
  Product5/1 -> Sum/2
  Product1/1 -> Sum/3
  Product2/1 -> Sum/4
  Product3/1 -> Sum/5
  Product4/1 -> Sum/6
  Transfer Fcn1/1 -> Transfer Fcn6/1
  Transfer Fcn6/1 -> Product5/1
  Transfer Fcn2/1 -> Transfer Fcn7/1
  Transfer Fcn7/1 -> Product1/1
  Transfer Fcn3/1 -> Transfer Fcn8/1
  Transfer Fcn8/1 -> Product2/1
  Transfer Fcn4/1 -> Transfer Fcn9/1
  Transfer Fcn9/1 -> Product3/1
  Transfer Fcn5/1 -> Transfer Fcn10/1
  Transfer Fcn10/1 -> Product4/1

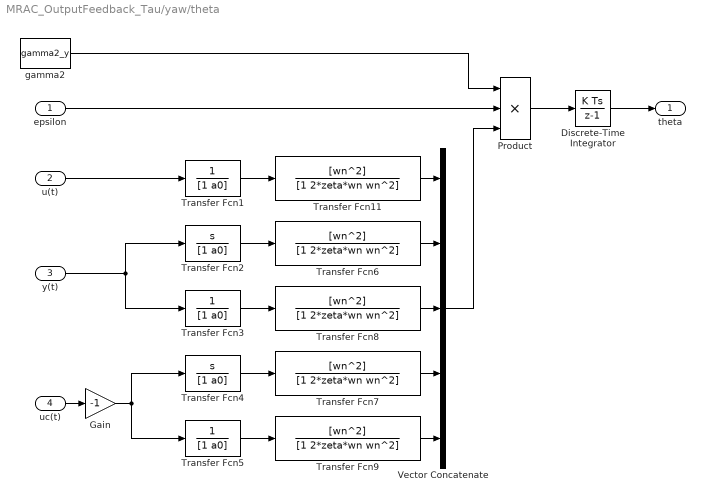
== system MRAC_OutputFeedback_Tau/yaw/theta ==
  epsilon : Inport
  u(t) : Inport  Port=2
  y(t) : Inport  Port=3
  uc(t) : Inport  Port=4
  Discrete-Time Integrator : DiscreteIntegrator  InitialCondition=theta_zero_y  InitialConditionSetting=State (most efficient)  SampleTime=-1  ICPrevOutput=DiscIntNeverNeededParam  ICPrevScaledInput=DiscIntNeverNeededParam
  Gain : Gain  Gain=-1
  Product : Product  Inputs=3
  Transfer Fcn1 : TransferFcn  Denominator=[1 a0]
  Transfer Fcn{6..9,11} (5 alike) : TransferFcn  Numerator=[wn^2]  Denominator=[1 2*zeta*wn wn^2]
  Transfer Fcn2 : TransferFcn  Numerator=[1 0]  Denominator=[1 a0]
  Transfer Fcn3 : TransferFcn  Denominator=[1 a0]
  Transfer Fcn4 : TransferFcn  Numerator=[1 0]  Denominator=[1 a0]
  Transfer Fcn5 : TransferFcn  Denominator=[1 a0]
  Vector Concatenate : Concatenate  NumInputs=5
  gamma2 : Constant  Value=gamma2_y
  theta : Outport
  wires:
  gamma2/1 -> Product/1
  epsilon/1 -> Product/2
  Discrete-Time Integrator/1 -> theta/1
  Product/1 -> Discrete-Time Integrator/1
  Transfer Fcn2/1 -> Transfer Fcn6/1
  Transfer Fcn4/1 -> Transfer Fcn7/1
  Transfer Fcn3/1 -> Transfer Fcn8/1
  Transfer Fcn5/1 -> Transfer Fcn9/1
  Transfer Fcn1/1 -> Transfer Fcn11/1
  u(t)/1 -> Transfer Fcn1/1
  Transfer Fcn9/1 -> Vector Concatenate/5
  Transfer Fcn7/1 -> Vector Concatenate/4
  Transfer Fcn8/1 -> Vector Concatenate/3
  Transfer Fcn6/1 -> Vector Concatenate/2
  Transfer Fcn11/1 -> Vector Concatenate/1
  y(t)/1 -> Transfer Fcn2/1, Transfer Fcn3/1
  uc(t)/1 -> Gain/1
  Gain/1 -> Transfer Fcn5/1, Transfer Fcn4/1
  Vector Concatenate/1 -> Product/3
